simulink model "MBD_Sources_Clock"  (R2021b)
settings: Solver=FixedStepDiscrete  StartTime=0.0  StopTime=10.0  FixedStep=0.01  RelTol=1e-3
settings Model: Creator=waleed.elshemy  LastModifiedBy=waleed.elshemy

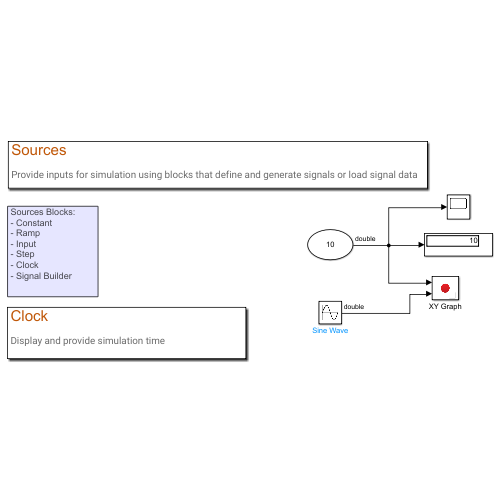
[thumbnail: Simulink's stored preview of the top-level diagram]
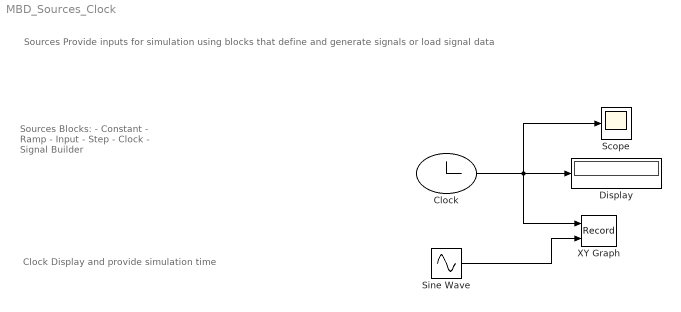
== system MBD_Sources_Clock ==
  note: Clock
      | Display and provide simulation time
  note: Sources
      | Provide inputs for simulation using blocks that define and generate signals or load signal data
  note: Sources Blocks:
      | - Constant
      | - Ramp
      | - Input
      | - Step
      | - Clock
      | - Signal Builder
  Clock : Clock
  Display : Display
  Scope : Scope
  Sine Wave : Sin  SampleTime=0
  XY Graph : Record  FileSettingsInternal="{\"entries\":[{\"content\":{\"excelSettings\":{\"content\":{},\"type\":\"Streamout.ExcelSettings\"}},\"type\":\"Streamout.FileSettingStorage\",\"uuid\":\"48ec0cd7-0070-417c-a57e-d2d4c765ff6c\"}],\"packageUris\":[\"http://schema.mathworks.com/mf0/streamout_blocks/R2020a\"],\"version\":\"1.0\"}"  Layout=[1 1]  SignalsInternal="{\"entries\":[{\"content\":{\"signals\":[{\"content\":{\"blockPath\":[\"MBD_Sources_Clock/XY Graph\"],\"channel\":[],\"dimensions\":[1],\"domain\":\"MBD_Sources_Clock/XY Graph\",\"lineColor\":\"#a2142f\",\"plots\":[1],\"port\":1,\"sid\":[\"\"],\"signalID\":181,\"signalName\":\"Clock\"},\"type\":\"RecordBlkView.Signal\",\"uuid\":\"faa79213-1fd8-4cfc-a22e-0d6501af0654\"},{\"content\":{\"blockPath\":[\"MBD_Sources_Clock/XY Graph\"],\"channel\":[],\"dimensions\":[1],\"domain\":\"MBD_Sources_Clock/XY Graph\",\"lineColor\":\"#139fff\",\"plots\":[1],\"port\":2,\"sid\":[\"\"],\"signalID\":185,\"signalName\":\"Sine Wave\"},\"type\":\"RecordBlkView.Signal\",\"uuid\":\"6e036d86-570d-48f0-a4c2-1e684efc3215\"}]},\"type\":\"RecordBlkView.InputSignals\",\"uuid\":\"51987374-00e9-4e97-bde1-4c7cd23f38c1\"}],\"packageUris\":[\"http://schema.mathworks.com/mf0/streamout_blocks/R2020a\"],\"version\":\"1.0\"}"  VisualizationBindings="{\"xyplotplugin\":{\"info\":[{\"series\":[{\"bindingParametersList\":[{\"parameter\":\"X-Axis\",\"signalID\":181,\"signalName\":\"Clock\"},{\"parameter\":\"Y-Axis\",\"signalID\":185,\"signalName\":\"Sine Wave\"}],\"seriesID\":13669}],\"subplotID\":1}]}}"  CompatibilityTag=XY
  wires:
  Clock/1 -> Scope/1, XY Graph/1, Display/1
  Sine Wave/1 -> XY Graph/2
